simulink model "balldetection"  (R2023a)
settings: Solver=VariableStepAuto  StartTime=0.0  StopTime=10.0  RelTol=1e-3
libraries: visionstatistics x1, imaqlib x1
settings Model: Creator=TIshX  LastModifiedBy=Flexible4

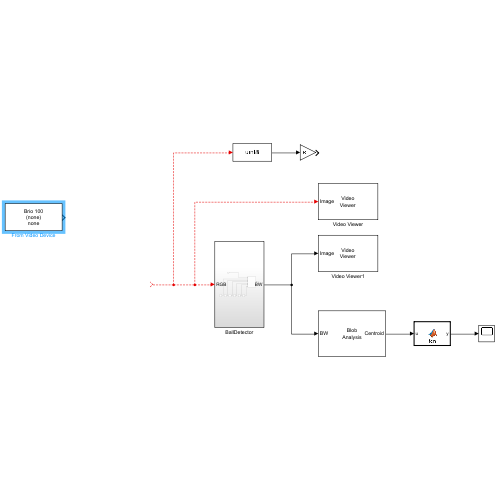
[thumbnail: Simulink's stored preview of the top-level diagram]
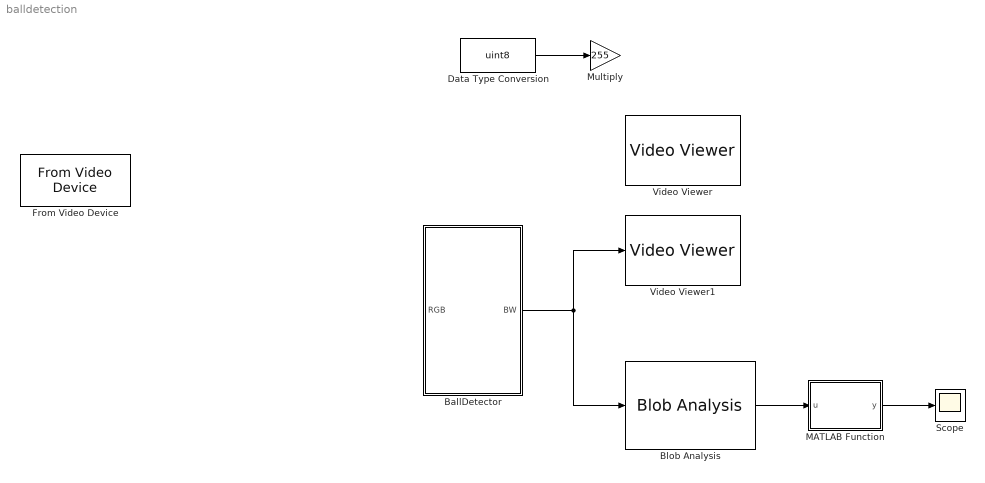
== system balldetection ==
  BallDetector : Subsystem
  Blob Analysis : visionstatistics/Blob Analysis  Tag=vipblks_row_conv  area=off  centroid=on  bBox=off  majorAxis=off  minorAxis=off  angle=off  eccentricity=off  equivDiameterSq=off  extent=off  perimeter=off  outDT=double  conn=8  isLabel=off  maxBlobs=50  warnIfNumBlobsExceeded=on  isCount=off  useMinArea=off  minArea=0  useMaxArea=off  maxArea=intmax('uint32')  excludeBorderBlob=off  isOutVarDim=off  isFill=on  fillValues=-1  roundingMode=Floor  overflowMode=off  prodOutputMode=Binary point scaling  prodOutputWordLength=32  prodOutputFracLength=16  accumMode=Binary point scaling  accumWordLength=32  accumFracLength=0  outputMode=Binary point scaling  outputWordLength=32  outputFracLength=16  firstCoeffMode=Binary point scaling  firstCoeffWordLength=16  firstCoeffFracLength=14  secondCoeffMode=Binary point scaling  secondCoeffWordLength=32  secondCoeffFracLength=16
  Data Type Conversion : DataTypeConversion  OutDataTypeStr=uint8  SaturateOnIntegerOverflow=off  RndMeth=Floor
  From Video Device : imaqlib/From Video Device  DeviceMenu=(none)  Device=winvideo 1 (Brio 100)  ObjConstructor=(none)  VideoFormatMenu=(none)  VideoFormat=(none)  VideoSource=none  ROIPosition=[0 0 576 1024]  EnableHWTrigger=off  SampleTime=1/30  OutputPortsMode=One multidimensional signal  DataType=single  CanDoHWTrigger=no  ReturnedColorSpace=rgb  BlockHandle=214.0002  ROIWidth=1024  ROIHeight=576  ROIColumn=0  ROIRow=0  EngXMLPath=C:\Program Files\MATLAB\R2023a\toolbox\imaq\imaq\private  DevXMLPath=C:\ProgramData\MATLAB\SupportPackages\R2023a\toolbox\imaq\supportpackages\genericvideo\adaptor\win64  EngLibPath=C:\Program Files\MATLAB\R2023a\toolbox\imaq\imaqblks\imaqmex\win64  ColorSpace=rgb  BayerSensorAlignment=grbg  ImaqMode=off
  MATLAB Function : MATLAB Function  TreatAsAtomicUnit=on
  Multiply : Gain  Gain=255
  Scope : Scope
  Video Viewer : VideoViewer  FigPos=[928 630 418 304]
  Video Viewer1 : VideoViewer  FigPos=[337 655 418 304]
  wires:
  ? -> Data Type Conversion/1, Video Viewer/1, BallDetector/1(RGB)
  BallDetector/1(BW) -> Blob Analysis/1, Video Viewer1/1
  Data Type Conversion/1 -> Multiply/1
  Blob Analysis/1 -> MATLAB Function/1(u)
  MATLAB Function/1(y) -> Scope/1

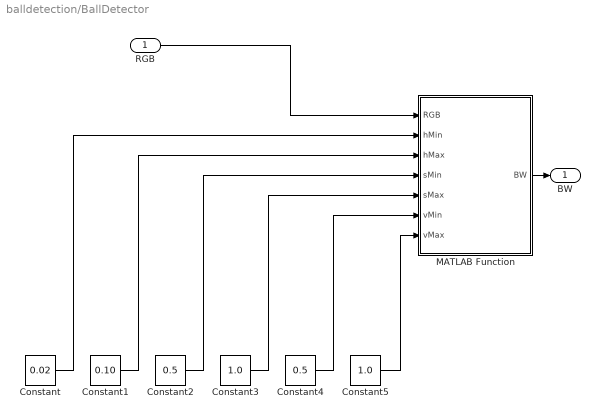
== system balldetection/BallDetector ==
  RGB : Inport
  Constant : Constant  Value=0.02
  Constant1 : Constant  Value=0.10
  Constant2 : Constant  Value=0.5
  Constant3 : Constant  Value=1.0
  Constant4 : Constant  Value=0.5
  Constant5 : Constant  Value=1.0
  MATLAB Function : MATLAB Function  TreatAsAtomicUnit=on
  BW : Outport
  wires:
  Constant4/1 -> MATLAB Function/6(vMin)
  MATLAB Function/1(BW) -> BW/1
  Constant3/1 -> MATLAB Function/5(sMax)
  Constant2/1 -> MATLAB Function/4(sMin)
  Constant/1 -> MATLAB Function/2(hMin)
  Constant1/1 -> MATLAB Function/3(hMax)
  Constant5/1 -> MATLAB Function/7(vMax)
  RGB/1 -> MATLAB Function/1(RGB)

== matlab function balldetection/MATLAB Function ==
  data: u input; y output
function y = fcn(u)

y = u(1);

== matlab function balldetection/BallDetector/MATLAB Function ==
  data: RGB input; BW output; hMin input; hMax input; sMin input; sMax input; vMin input; vMax input
function BW = detectBall(RGB, hMin, hMax, sMin, sMax, vMin, vMax)
    % HSVに変換
    I = rgb2hsv(RGB);
    
    % マスク作成（閾値は外部から）
    BW = (I(:,:,1) >= hMin) & (I(:,:,1) <= hMax) & ...
         (I(:,:,2) >= sMin) & (I(:,:,2) <= sMax) & ...
         (I(:,:,3) >= vMin) & (I(:,:,3) <= vMax);
end
